simulink model "gm_tutorial1_1_ref"  (R2020b)
settings: Solver=FixedStepDiscrete  StartTime=0.0  StopTime=simulation_stop_time  RelTol=1e-3
undefined symbols (not defined in the file or in its folder): sample_time
settings Model: Creator=yixingli  LastModifiedBy=harsh
settings DataIOCC: LimitDataPoints=on  SaveOutput=off  SignalLogging=off  SaveTime=off
settings OptimizationCC: BlockReduction=off  ConditionallyExecuteInputs=off  DefaultParameterBehavior=Inlined  OptimizeBlockIOStorage=off  ExpressionDepthLimit=2147483647
settings DebuggingCC: AlgebraicLoopMsg=error  UnderspecifiedInitializationDetection=Classic  MergeDetectMultiDrivingBlocksExec=none  InheritedTsInSrcMsg=none  SingleTaskRateTransMsg=error  ParameterPrecisionLossMsg=none  AllowSymbolicDim=off  StateNameClashWarn=warning  StrictBusMsg=ErrorOnBusTreatedAsVector  SFUnexpectedBacktrackingDiag=warning  SFNoUnconditionalDefaultTransitionDiag=warning  SFExecutionAtInitializationDiag=none  ArithmeticOperatorsInVariantConditions=warning
settings HardwareCC: ProdBitPerPointer=32  ProdBitPerSizeT=32  ProdBitPerPtrDiffT=32  ProdLargestAtomicFloat=None  ProdIntDivRoundTo=Undefined  ProdEndianess=Unspecified  ProdWordSize=32  ProdHWDeviceType=ASIC/FPGA->ASIC/FPGA  TargetBitPerPointer=64  TargetBitPerSizeT=64  TargetBitPerPtrDiffT=64  TargetLongLongMode=on  TargetIntDivRoundTo=Zero  TargetEndianess=LittleEndian  TargetWordSize=64  TargetHWDeviceType=Generic->Custom  ProdEqTarget=off
settings SFSimCC: SimUseLocalCustomCode=off  CustomCodeUndefinedFunction=UseInterfaceOnly
settings RTWCC: Description=SystemVerilog DPI Component Generator  SystemTargetFile=systemverilog_dpi_grt.tlc  TemplateMakefile=systemverilog_dpi_grt_default_tmf  RTWVerbose=off  RTWUseLocalCustomCode=off  BuildConfiguration=Faster Runs
settings CodeAppCC: MaxIdLength=256  StateflowObjectComments=on
settings DPIGRTTargetCC: TargetFcnLib=ansi_tfl_table_tmw.mat  GenFloatMathFcnCalls=NOT IN USE  TargetLangStandard=C89/C90 (ANSI)  CodeReplacementLibrary=None  UtilityFuncGeneration=Auto  MultiwordTypeDef=System defined  MultiwordLength=2048  DynamicStringBufferSize=256  GenerateFullHeader=on  InferredTypesCompatibility=off  GenerateSampleERTMain=off  GenerateTestInterfaces=off  ModelReferenceCompliant=on  ParMdlRefBuildCompliant=on  CompOptLevelCompliant=off  ConcurrentExecutionCompliant=off  IncludeMdlTerminateFcn=on  CombineOutputUpdateFcns=off  CombineSignalStateStructs=on  GroupInternalDataByFunction=off  SuppressErrorStatus=off  IncludeFileDelimiter=Auto  ERTCustomFileBanners=off  SupportAbsoluteTime=on  LogVarNameModifier=rt_  MatFileLogging=off  CodeInterfacePackaging=Reusable function  PurelyIntegerCode=off  SupportNonFinite=on  SupportComplex=on  SupportContinuousTime=on  SupportNonInlinedSFcns=on  RemoveDisableFunc=off  RemoveResetFunc=off  SupportVariableSizeSignals=off  ParenthesesLevel=Nominal  CastingMode=Nominal  MATLABClassNameForMDSCustomization=Simulink.SoftwareTarget.TargetSpecificTriggerConfigurationBase  ModelStepFunctionPrototypeControlCompliant=off  CPPClassGenCompliant=off  AutosarCompliant=off  MDXCompliant=off  GRTInterface=off  GenerateAllocFcn=on  UseToolchainInfoCompliant=on  GenerateSharedConstants=on  CoderGroups=[]  AccessMethods=[]  LookupTableObjectStructAxisOrder=1,2,3,4,...  LUTObjectStructOrderExplicitValues=Size,Breakpoints,Table  LUTObjectStructOrderEvenSpacing=Size,Breakpoints,Table  ArrayLayout=Column-major  UnsupportedSFcnMsg=error  ERTHeaderFileRootName=$R$E  ERTSourceFileRootName=$R$E  ERTDataFileRootName=$R_data  RTWCAPISignals=on  RTWCAPIParams=off  RTWCAPIStates=off  RTWCAPIRootIO=off  ExtMode=off  ExtModeTransport=0  ExtModeStaticAlloc=off  ExtModeStaticAllocSize=1000000  ExtModeTesting=off  ExtModeMexFile=ext_comm  GenerateASAP2=off  MultiInstanceErrorCode=Error  DPICustomizeSystemVerilogCode=on  DPISystemVerilogTemplate=hdlverifier_dpitb_template.vgt  DPIReportRunTimeError=off  DPIRunTimeErrorSeverity=Fatal  DPIGenerateTestBench=off  DPITestBenchSimulator=Mentor Graphics Questasim  DPITestPointAccessFcnInterface=None  DPIFixedPointDataType=CompatibleCType  DPIPortConnection=Port list  DPICompositeDataType=Flattened
settings ConfigComp: CovScope=ReferencedModels  CovMetricSettings=dw  CovSaveCumulativeToWorkspaceVar=on  CovSaveSingleToWorkspaceVar=on  CovExternalEMLEnable=off  CovSFcnEnable=off

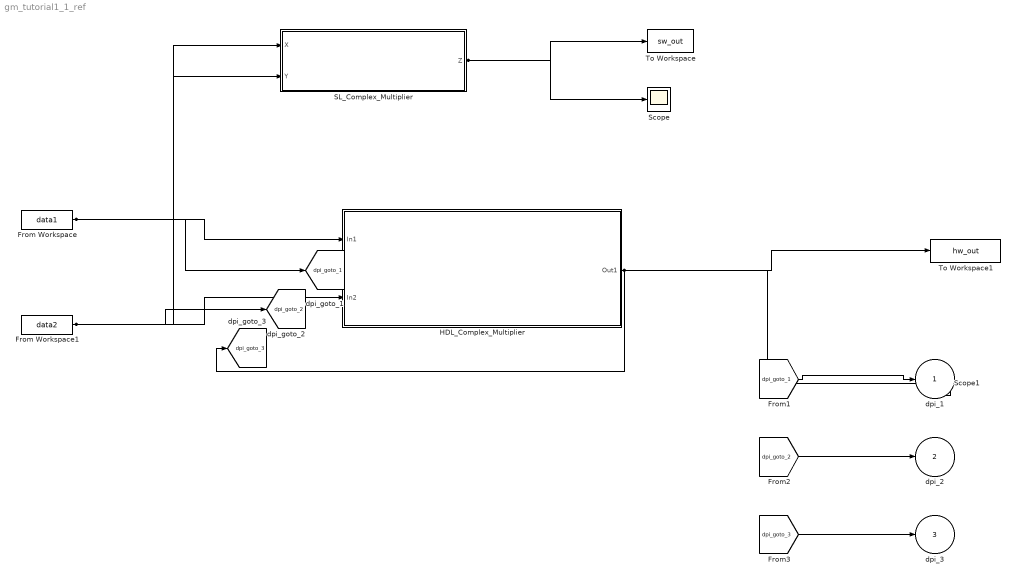
== system gm_tutorial1_1_ref ==
  From Workspace : FromWorkspace  VariableName=data1  SampleTime=sample_time  Interpolate=off  OutputAfterFinalValue=Setting to zero
  From Workspace1 : FromWorkspace  VariableName=data2  SampleTime=sample_time  Interpolate=off  OutputAfterFinalValue=Setting to zero
  HDL_Complex_Multiplier : Subsystem
  SL_Complex_Multiplier : Subsystem
  Scope : Scope
  Scope1 : Scope
  To Workspace : ToWorkspace  VariableName=sw_out  SaveFormat=Structure With Time  SampleTime=-1
  To Workspace1 : ToWorkspace  VariableName=hw_out  SaveFormat=Structure With Time  SampleTime=-1
  dpi_1 : Outport
  dpi_2 : Outport  Port=2
  dpi_3 : Outport  Port=3
  tag scope: dpi_goto_1=global, dpi_goto_2=global, dpi_goto_3=global
  wires:
  SL_Complex_Multiplier/1(Z) -> To Workspace/1, Scope/1
  From Workspace/1 -> HDL_Complex_Multiplier/1(In1), SL_Complex_Multiplier/1(X), [dpi_goto_1]
  From Workspace1/1 -> HDL_Complex_Multiplier/2(In2), SL_Complex_Multiplier/2(Y), [dpi_goto_2]
  HDL_Complex_Multiplier/1(Out1) -> Scope1/1, To Workspace1/1, [dpi_goto_3]
  [dpi_goto_1] -> dpi_1/1
  [dpi_goto_2] -> dpi_2/1
  [dpi_goto_3] -> dpi_3/1

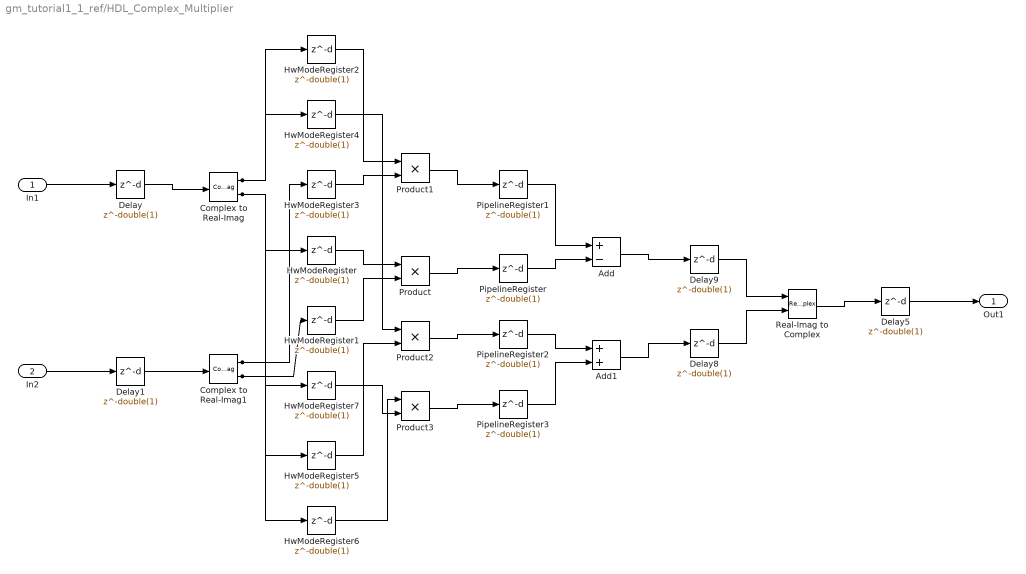
== system gm_tutorial1_1_ref/HDL_Complex_Multiplier ==
  In1 : Inport  OutDataTypeStr=fixdt(1, 12, 8)  PortDimensions=1  SampleTime=1e-06
      settings: SignalType=complex
  In2 : Inport  Port=2  OutDataTypeStr=fixdt(1, 12, 8)  PortDimensions=1  SampleTime=1e-06
      settings: SignalType=complex
  Add : Sum  Inputs=+-  AccumDataTypeStr=fixdt(1, 25, 16)  OutDataTypeStr=fixdt(1, 25, 16)  SampleTime=1e-06
  Add1 : Sum  AccumDataTypeStr=fixdt(1, 25, 16)  OutDataTypeStr=fixdt(1, 25, 16)  SampleTime=1e-06
  Complex to Real-Imag : ComplexToRealImag  SampleTime=1e-06
  Complex to Real-Imag1 : ComplexToRealImag  SampleTime=1e-06
  Delay{,1,5,8..9} (5 alike) : Delay  DelayLength=double(1)  InitialCondition=0  SampleTime=1e-06
  HwModeRegister{,1..7} (8 alike) : Delay  DelayLength=double(1)  InitialCondition=0  SampleTime=1e-06
  PipelineRegister{,1..3} (4 alike) : Delay  DelayLength=double(1)  InitialCondition=0  SampleTime=1e-06
  Product{,1..3} (4 alike) : Product  Inputs=**  OutDataTypeStr=fixdt(1, 24, 16)  SampleTime=1e-06
  Real-Imag to Complex : RealImagToComplex  ConstantPart="fi(0,1,25,16,\"hex\",\"0000000\")"  SampleTime=1e-06
  Out1 : Outport
  wires:
  HwModeRegister7/1 -> Product3/2
  HwModeRegister6/1 -> Product3/1
  Product3/1 -> PipelineRegister3/1
  HwModeRegister5/1 -> Product2/2
  HwModeRegister4/1 -> Product2/1
  Product2/1 -> PipelineRegister2/1
  HwModeRegister3/1 -> Product1/2
  HwModeRegister2/1 -> Product1/1
  Product1/1 -> PipelineRegister1/1
  HwModeRegister1/1 -> Product/2
  HwModeRegister/1 -> Product/1
  Product/1 -> PipelineRegister/1
  Real-Imag to Complex/1 -> Delay5/1
  PipelineRegister3/1 -> Add1/2
  PipelineRegister2/1 -> Add1/1
  PipelineRegister1/1 -> Add/1
  PipelineRegister/1 -> Add/2
  Delay9/1 -> Real-Imag to Complex/1
  Delay8/1 -> Real-Imag to Complex/2
  Delay5/1 -> Out1/1
  Delay1/1 -> Complex to Real-Imag1/1
  Delay/1 -> Complex to Real-Imag/1
  Complex to Real-Imag1/2 -> HwModeRegister5/1, HwModeRegister1/1
  Complex to Real-Imag1/1 -> HwModeRegister6/1, HwModeRegister3/1
  Complex to Real-Imag/2 -> HwModeRegister7/1, HwModeRegister/1
  Complex to Real-Imag/1 -> HwModeRegister4/1, HwModeRegister2/1
  Add1/1 -> Delay8/1
  Add/1 -> Delay9/1
  In2/1 -> Delay1/1
  In1/1 -> Delay/1

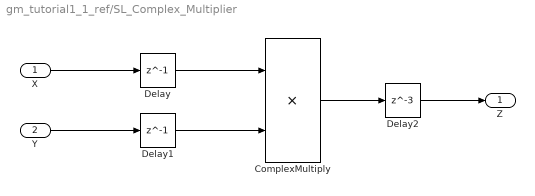
== system gm_tutorial1_1_ref/SL_Complex_Multiplier ==
  X : Inport
  Y : Inport  Port=2
  ComplexMultiply : Product
  Delay : Delay  DelayLength=1  InitialCondition=0
  Delay1 : Delay  DelayLength=1  InitialCondition=0
  Delay2 : Delay  DelayLength=3  InitialCondition=0
  Z : Outport  VectorParamsAs1DForOutWhenUnconnected=off
  wires:
  ComplexMultiply/1 -> Delay2/1
  X/1 -> Delay/1
  Y/1 -> Delay1/1
  Delay1/1 -> ComplexMultiply/2
  Delay/1 -> ComplexMultiply/1
  Delay2/1 -> Z/1
